simulink model "controladorLQRSwitch"  (Simulink 7.9)
settings: Solver=ode45  StartTime=0.0  StopTime=10  MaxStep=0.03  MinStep=0.01  RelTol=1e-3
values from neighbouring files (symbols this model uses):
  K = lqr(A,B,Q,R)    [LQR.m]    (also in bestQ.m = setK_lqr(Q_i); graficosPenduloReal.m = setK_lqr(Q_optimo))
undefined symbols (not defined in the file or in its folder): globalState
settings Model: Creator=Daniel  LastModifiedBy=root
settings SolverCC: InitialStep=0.01
settings DebuggingCC: FcnCallInpInsideContextMsg=Use local settings  StrictBusMsg=Warning
settings SFSimCC: SimParseCustomCode=off
settings GRTTargetCC: CombineOutputUpdateFcns=off  GRTInterface=on

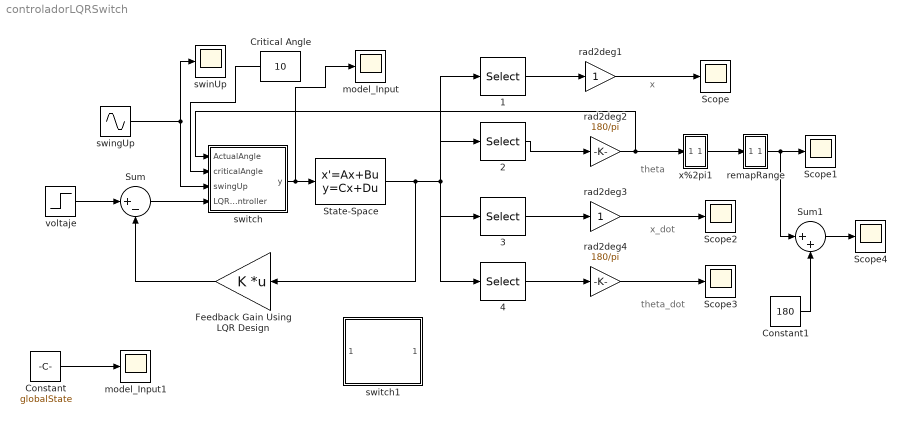
== system controladorLQRSwitch ==
  note: x
  note: theta
  note: theta_dot
  note: x_dot
  " 1" : Selector  InputPortWidth=4  IndexOptions=Index vector (dialog)  Indices=1  OutputSizes=1
  " 2" : Selector  InputPortWidth=4  IndexOptions=Index vector (dialog)  Indices=2  OutputSizes=1
  " 3" : Selector  InputPortWidth=4  IndexOptions=Index vector (dialog)  Indices=3  OutputSizes=1
  " 4" : Selector  InputPortWidth=4  IndexOptions=Index vector (dialog)  Indices=4  OutputSizes=1
  Constant : Constant  Value=globalState
  Constant1 : Constant  Value=180
  Critical Angle : Constant  Value=10
  Feedback Gain Using LQR Design : Gain  Gain=K  Multiplication=Matrix(K*u) (u vector)
  Scope{,1..4} (5 alike) : Scope
      Scope1 settings: SaveName=thetaLineal
      Scope2 settings: SaveName=ScopeData2
      Scope3 settings: SaveName=ScopeData3
      Scope4 settings: SaveName=thetaLineal1
  State-Space : StateSpace  A="[0 0 1 0; 0 0 0 1; 0 0.5401 -0.7235 0; 0  14.955 -0.9854 0]"  B="[0  ;0 ;2.2747 ;3.0978]"  C=eye(4)  D=[0;0;0;0]  X0=[0;180*pi/180;0;0]
  Sum : Sum  Inputs=|+-
  Sum1 : Sum  Inputs=|++
  model_Input : Scope
  model_Input1 : Scope
      settings: SaveName=ScopeData5
  rad2deg1 : Gain  SaturateOnIntegerOverflow=on  OutDataTypeStr=Inherit: Same as input  ParamDataTypeStr=Inherit: Same as input
  rad2deg2 : Gain  Gain=180/pi  SaturateOnIntegerOverflow=on  OutDataTypeStr=Inherit: Same as input  ParamDataTypeStr=Inherit: Same as input
  rad2deg3 : Gain  SaturateOnIntegerOverflow=on  OutDataTypeStr=Inherit: Same as input  ParamDataTypeStr=Inherit: Same as input
  rad2deg4 : Gain  Gain=180/pi  SaturateOnIntegerOverflow=on  OutDataTypeStr=Inherit: Same as input  ParamDataTypeStr=Inherit: Same as input
  remapRange : MATLAB Function  TreatAsAtomicUnit=on
  swinUp : Scope
      settings: SaveName=ScopeData4
  swingUp : Sin  Frequency=20  SampleTime=0
  switch : MATLAB Function  TreatAsAtomicUnit=on
  switch1 : MATLAB Function  TreatAsAtomicUnit=on
  voltaje : Step  Time=0  After=0  SampleTime=0
  x%2pi1 : MATLAB Function  TreatAsAtomicUnit=on
  wires:
  " 1"/1 -> rad2deg1/1
  " 2"/1 -> rad2deg2/1
  rad2deg4/1 -> Scope3/1
  rad2deg2/1 -> x%2pi1/1(u), switch/1(ActualAngle)
  rad2deg1/1 -> Scope/1
  State-Space/1 -> " 1"/1, " 3"/1, " 2"/1, " 4"/1, Feedback Gain Using LQR Design/1
  " 4"/1 -> rad2deg4/1
  voltaje/1 -> Sum/1
  swingUp/1 -> swinUp/1, switch/3(swingUp)
  Critical Angle/1 -> switch/2(criticalAngle)
  " 3"/1 -> rad2deg3/1
  rad2deg3/1 -> Scope2/1
  x%2pi1/1(y) -> remapRange/1(value)
  remapRange/1(y) -> Scope1/1, Sum1/1
  Constant/1 -> model_Input1/1
  switch/1(y) -> State-Space/1, model_Input/1
  Sum/1 -> switch/4(LQRcontroller)
  Constant1/1 -> Sum1/2
  Sum1/1 -> Scope4/1
  Feedback Gain Using LQR Design/1 -> Sum/2

== matlab function switch ==
  data: y output double; ActualAngle input double; criticalAngle input double; swingUp input double; LQRcontroller input double
function y = fcn(ActualAngle, criticalAngle, swingUp, LQRcontroller)
%
if (ActualAngle < criticalAngle)
    y = swingUp;
else
    y = LQRcontroller;
end
end

== matlab function switch1 ==
  data: varUpdate input double; varUpdated output double
function varUpdated  = globalHandler(varUpdate)
%
    if(varUpdate == 1)
        var =  1;
    else
        var = 0;
    end
    if (varUpdate==1)
        varUpdated = 1;
    else
        varUpdated = 0;
    end
end

== matlab function remapRange ==
  data: value input double; y output double
function y = remapRange(value)
    scaleFactor = 1;
    if (value>180*scaleFactor)
        %constants
        fromLow = 181*scaleFactor;
        fromHigh = 360*scaleFactor;
        toLow = -179*scaleFactor;
        toHigh = 0*scaleFactor;
        %calculations
        new_range = toHigh-toLow;
        old_range = fromHigh - fromLow;
        new_value = (new_range/old_range)*(value-fromLow)+toLow;
        y = new_value;
    else
        y = value;
    end
        
end

== matlab function x%2pi1 ==
  data: u input double; y output double
function y = fcn(u)
%#codegen

    y = mod(u,360);
end
